simulink model "v_5_IHA_NEW_Plant"  (R2020b)
settings: Solver=VariableStepAuto  StartTime=0.0  StopTime=10  RelTol=1e-3  EnableMultiTasking=on
InitFcn:
  | variables;
values from neighbouring files (symbols this model uses):
  b = 54.2e-6    (= 5.42e-05)    [variables.m]
  d = 1.1e-6    (= 1.1e-06)    [variables.m]
  g = 9.81    [variables.m]
  Ixx = 8.1e-3    (= 0.0081)    [variables.m]
  Iyy = 8.1e-3    (= 0.0081)    [variables.m]
  Izz = 14.2e-3    (= 0.0142)    [variables.m]
  Jr = 104e-6    (= 0.000104)    [variables.m]
  L = 0.24    [variables.m]
  m = 1.0    (= 1)    [variables.m]
  Phi_D = 5    [variables.m]
  Phi_P = 30    [variables.m]
  Psi_D = 5    [variables.m]
  Psi_P = 30    [variables.m]
  Theta_D = 5    [variables.m]
  Theta_P = 30    [variables.m]
  Ts = 0.01    [find_metrics_DQN.m]    (also in v_5_IHA_NEW_Plant_For_DDPG.m; v_5_IHA_NEW_Plant_For_DQN.m)
  Z_D = 12    [variables.m]
  Z_P = 40    [variables.m]
undefined symbols (not defined in the file or in its folder): DiscIntNeverNeededParam
libraries: rllib x4, dspswit3 x4, simulink x3
settings Model: Creator=RafadanTayfa  LastModifiedBy=RafadanTayfa
settings SolverCC: ZeroCrossAlgorithm=Adaptive

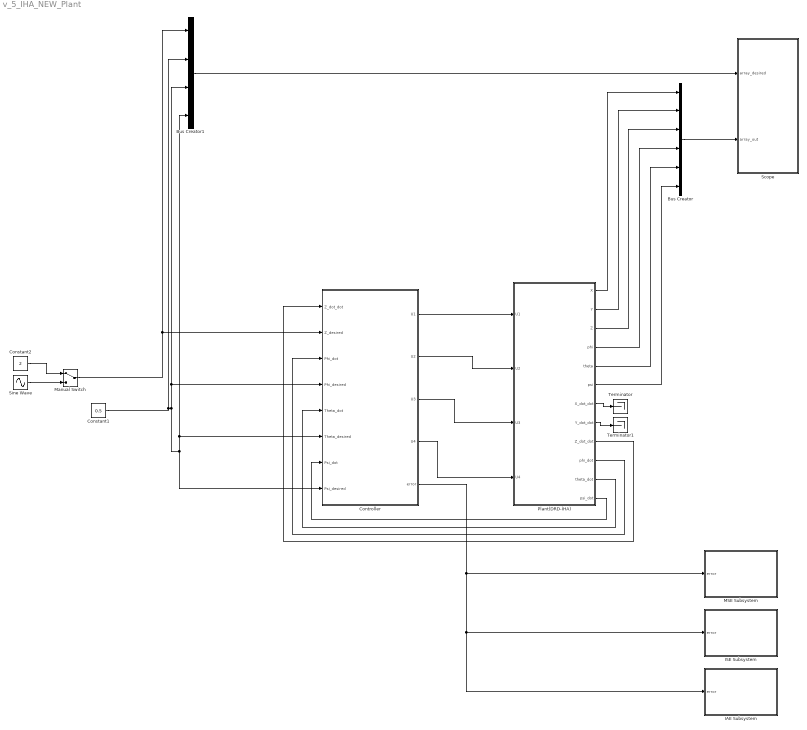
== system v_5_IHA_NEW_Plant ==
  Bus Creator : BusCreator  Inputs=6
  Bus Creator1 : BusCreator  Inputs=4
  Constant1 : Constant  Value=0.5
  Constant2 : Constant  Value=2
  Controller : Subsystem
  IAE Subsystem : Subsystem
  ISE Subsystem : Subsystem
  MSE Subsystem : Subsystem
  Manual Switch : ManualSwitch
  Plant(DRD-İHA) : Subsystem
  Scope : Subsystem
  Sine Wave : Sin  Bias=6  Frequency=pi/2  SampleTime=0
  Terminator : Terminator
  Terminator1 : Terminator
  wires:
  Plant(DRD-İHA)/7(X_dot_dot) -> Terminator/1
  Controller/4(U4) -> Plant(DRD-İHA)/4(U4)
  Controller/3(U3) -> Plant(DRD-İHA)/3(U3)
  Controller/2(U2) -> Plant(DRD-İHA)/2(U2)
  Controller/1(U1) -> Plant(DRD-İHA)/1("U1 ")
  Plant(DRD-İHA)/12(psi_dot) -> Controller/7(Psi_dot)
  Plant(DRD-İHA)/10(phi_dot) -> Controller/3(Phi_dot)
  Plant(DRD-İHA)/11(theta_dot) -> Controller/5(Theta_dot)
  Plant(DRD-İHA)/2(Y) -> Bus Creator/2
  Plant(DRD-İHA)/1(X) -> Bus Creator/1
  Plant(DRD-İHA)/3(Z) -> Bus Creator/3
  Plant(DRD-İHA)/4(phi) -> Bus Creator/4
  Plant(DRD-İHA)/5(theta) -> Bus Creator/5
  Plant(DRD-İHA)/6(psi) -> Bus Creator/6
  Manual Switch/1 -> Bus Creator1/1, Controller/2(Z_desired)
  Constant1/1 -> Bus Creator1/2, Controller/4(Phi_desired), Bus Creator1/3, Controller/6(Theta_desired), Bus Creator1/4, Controller/8(Psi_desired)
  Bus Creator1/1 -> Scope/1(array_desired)
  Bus Creator/1 -> Scope/2(array_out)
  Plant(DRD-İHA)/9(Z_dot_dot) -> Controller/1("Z_dot_dot ")
  Plant(DRD-İHA)/8(Y_dot_dot) -> Terminator1/1
  Controller/5(error) -> MSE Subsystem/1(error), IAE Subsystem/1(error), ISE Subsystem/1(error)
  Constant2/1 -> Manual Switch/1
  Sine Wave/1 -> Manual Switch/2

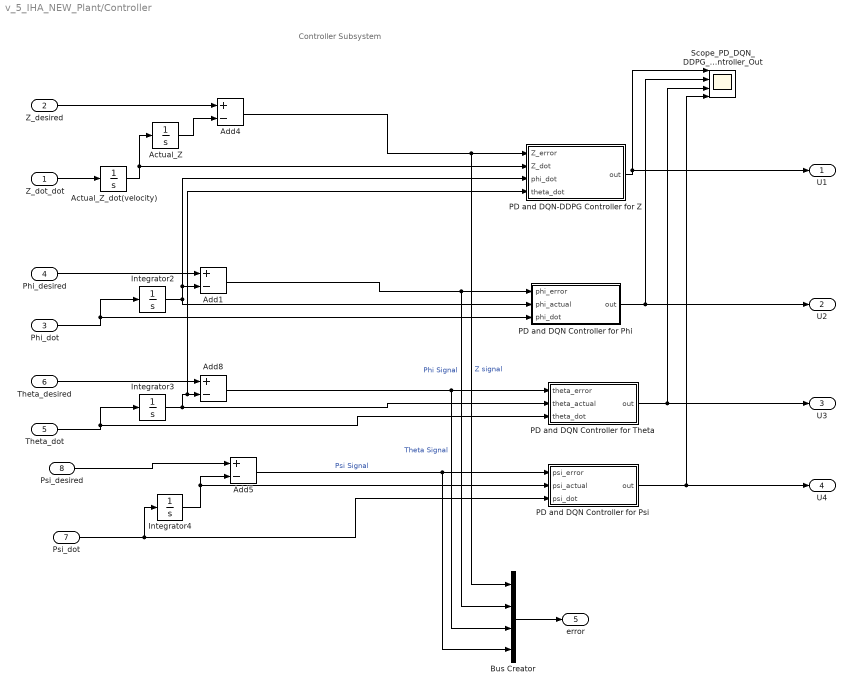
== system v_5_IHA_NEW_Plant/Controller ==
  note: Controller Subsystem
  "Z_dot_dot " : Inport
  Z_desired : Inport  Port=2
  Phi_dot : Inport  Port=3
  Phi_desired : Inport  Port=4
  Theta_dot : Inport  Port=5
  Theta_desired : Inport  Port=6
  Psi_dot : Inport  Port=7
  Psi_desired : Inport  Port=8
  Actual_Z : Integrator  LimitOutput=on  UpperSaturationLimit=800  LowerSaturationLimit=0  ZeroCross=off
  Actual_Z_dot(velocity) : Integrator  ZeroCross=off
  Add{1,4..5,8} (4 alike) : Sum  Inputs=+-
  Bus Creator : BusCreator  Inputs=4
  Integrator2 : Integrator  WrapState=on  ZeroCross=off
  Integrator3 : Integrator  WrapState=on  ZeroCross=off
  Integrator4 : Integrator  WrapState=on  ZeroCross=off
  PD and DQN Controller for Phi : Subsystem
  PD and DQN Controller for Psi : Subsystem
  PD and DQN Controller for Theta : Subsystem
  PD and DQN-DDPG Controller for Z : Subsystem
  Scope_PD_DQN_DDPG_Controller_Out : Scope  NumInputPorts=4
  U1 : Outport
  U2 : Outport  Port=2
  U3 : Outport  Port=3
  U4 : Outport  Port=4
  error : Outport  Port=5
  wires:
  Phi_desired/1 -> Add1/1
  "Z_dot_dot "/1 -> Actual_Z_dot(velocity)/1
  Actual_Z_dot(velocity)/1 -> Actual_Z/1, PD and DQN-DDPG Controller for Z/2(Z_dot)
  Integrator2/1 -> PD and DQN Controller for Phi/2(phi_actual), PD and DQN-DDPG Controller for Z/3(phi_dot), Add1/2
  Add1/1 -> Bus Creator/2, PD and DQN Controller for Phi/1(phi_error)  "Phi Signal"
  Integrator3/1 -> PD and DQN-DDPG Controller for Z/4(theta_dot), Add8/2, PD and DQN Controller for Theta/2(theta_actual)
  Theta_desired/1 -> Add8/1
  Theta_dot/1 -> PD and DQN Controller for Theta/3(theta_dot), Integrator3/1
  Add8/1 -> Bus Creator/3, PD and DQN Controller for Theta/1(theta_error)  "Theta Signal"
  Actual_Z/1 -> Add4/2
  Z_desired/1 -> Add4/1
  Psi_desired/1 -> Add5/1
  Add5/1 -> Bus Creator/4, PD and DQN Controller for Psi/1(psi_error)  "Psi Signal"
  Add4/1 -> Bus Creator/1, PD and DQN-DDPG Controller for Z/1(Z_error)  "Z signal"
  PD and DQN-DDPG Controller for Z/1(out) -> Scope_PD_DQN_DDPG_Controller_Out/1, U1/1
  Phi_dot/1 -> PD and DQN Controller for Phi/3(phi_dot), Integrator2/1
  Psi_dot/1 -> Integrator4/1, PD and DQN Controller for Psi/3(psi_dot)
  Integrator4/1 -> PD and DQN Controller for Psi/2(psi_actual), Add5/2
  Bus Creator/1 -> error/1
  PD and DQN Controller for Phi/1(out) -> U2/1, Scope_PD_DQN_DDPG_Controller_Out/2
  PD and DQN Controller for Theta/1(out) -> U3/1, Scope_PD_DQN_DDPG_Controller_Out/3
  PD and DQN Controller for Psi/1(out) -> U4/1, Scope_PD_DQN_DDPG_Controller_Out/4

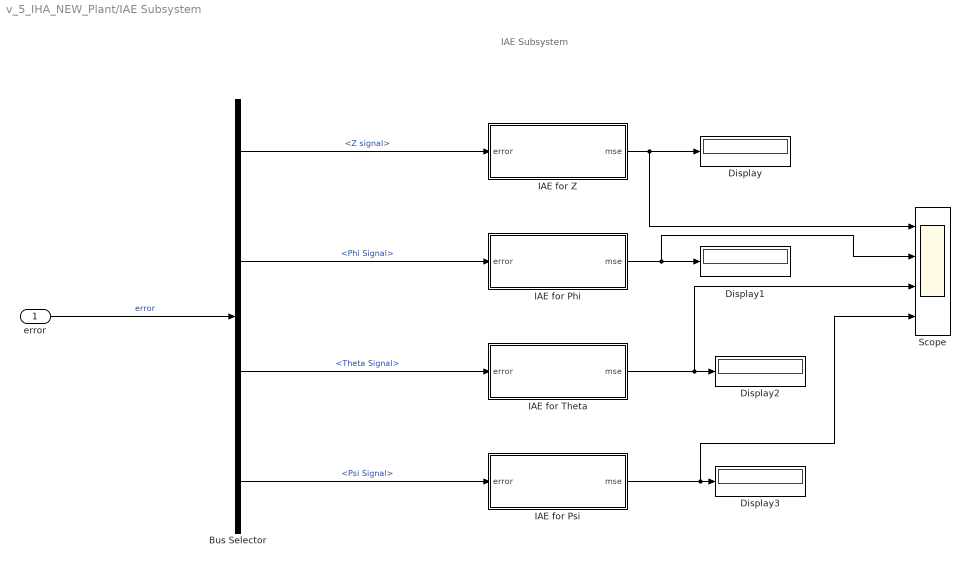
== system v_5_IHA_NEW_Plant/IAE Subsystem ==
  note: IAE Subsystem
  error : Inport
  Bus Selector : BusSelector  OutputSignals=Z signal,Phi Signal,Theta Signal,Psi Signal
  Display{,1..3} (4 alike) : Display
  IAE for Phi : Subsystem
  IAE for Psi : Subsystem
  IAE for Theta : Subsystem
  IAE for Z : Subsystem
  Scope : Scope  NumInputPorts=4
  wires:
  IAE for Z/1(mse) -> Scope/1, Display/1
  error/1 -> Bus Selector/1  "error"
  Bus Selector/1 -> IAE for Z/1(error)  "<Z signal>"
  IAE for Phi/1(mse) -> Scope/2, Display1/1
  Bus Selector/2 -> IAE for Phi/1(error)  "<Phi Signal>"
  Bus Selector/3 -> IAE for Theta/1(error)  "<Theta Signal>"
  Bus Selector/4 -> IAE for Psi/1(error)  "<Psi Signal>"
  IAE for Theta/1(mse) -> Scope/3, Display2/1
  IAE for Psi/1(mse) -> Scope/4, Display3/1

== system v_5_IHA_NEW_Plant/ISE Subsystem ==
  note: ISE Subsystem
  error : Inport
  Bus Selector : BusSelector  OutputSignals=Z signal,Phi Signal,Theta Signal,Psi Signal
  Display{,1..3} (4 alike) : Display
  ISE for Phi : Subsystem
  ISE for Psi : Subsystem
  ISE for Theta : Subsystem
  ISE for Z : Subsystem
  Scope : Scope  NumInputPorts=4
  wires:
  ISE for Psi/1(mse) -> Display3/1, Scope/4
  ISE for Theta/1(mse) -> Display2/1, Scope/3
  Bus Selector/4 -> ISE for Psi/1(error)  "<Psi Signal>"
  Bus Selector/3 -> ISE for Theta/1(error)  "<Theta Signal>"
  Bus Selector/2 -> ISE for Phi/1(error)  "<Phi Signal>"
  ISE for Phi/1(mse) -> Display1/1, Scope/2
  Bus Selector/1 -> ISE for Z/1(error)  "<Z signal>"
  error/1 -> Bus Selector/1  "error"
  ISE for Z/1(mse) -> Display/1, Scope/1

== system v_5_IHA_NEW_Plant/MSE Subsystem ==
  note: MSE Subsystem
  error : Inport
  Bus Selector : BusSelector  OutputSignals=Z signal,Phi Signal,Theta Signal,Psi Signal
  Display{,1..3} (4 alike) : Display
  MSE for Phi : Subsystem
  MSE for Psi : Subsystem
  MSE for Theta : Subsystem
  MSE for Z : Subsystem
  Scope : Scope  NumInputPorts=4
  wires:
  MSE for Z/1(mse) -> Scope/1, Display/1
  error/1 -> Bus Selector/1  "error"
  Bus Selector/1 -> MSE for Z/1(error)  "<Z signal>"
  MSE for Phi/1(mse) -> Scope/2, Display1/1
  Bus Selector/2 -> MSE for Phi/1(error)  "<Phi Signal>"
  Bus Selector/3 -> MSE for Theta/1(error)  "<Theta Signal>"
  Bus Selector/4 -> MSE for Psi/1(error)  "<Psi Signal>"
  MSE for Theta/1(mse) -> Scope/3, Display2/1
  MSE for Psi/1(mse) -> Scope/4, Display3/1

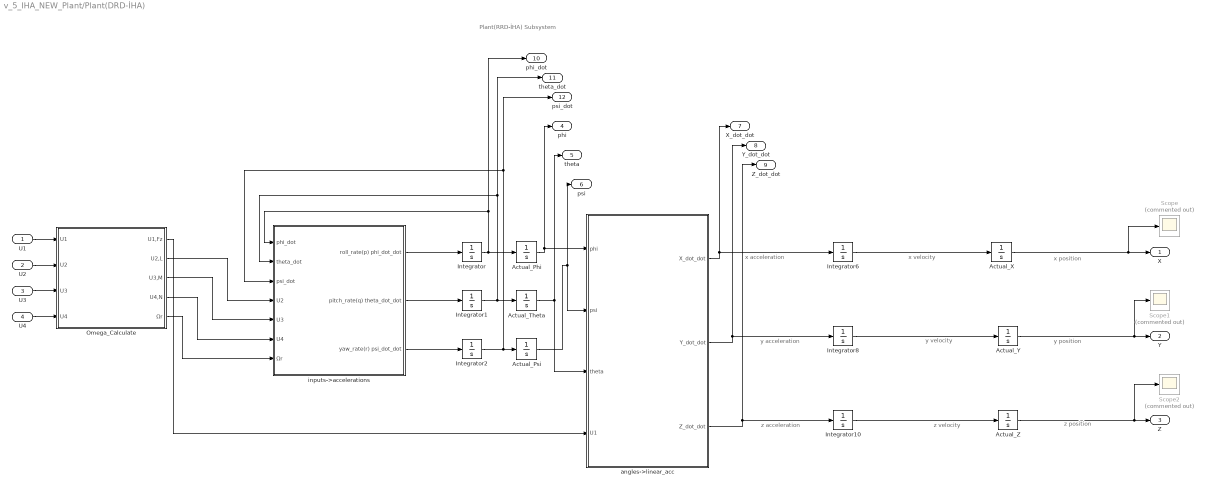
== system v_5_IHA_NEW_Plant/Plant(DRD-İHA) ==
  note: Plant(RRD-İHA) Subsystem
  note: z position
  note: y position
  note: x position
  note: z velocity
  note: y velocity
  note: x velocity
  note: z acceleration
  note: y acceleration
  note: x acceleration
  "U1 " : Inport
  U2 : Inport  Port=2
  U3 : Inport  Port=3
  U4 : Inport  Port=4
  Actual_Phi : Integrator  WrapState=on  ZeroCross=off
  Actual_Psi : Integrator  WrapState=on  ZeroCross=off
  Actual_Theta : Integrator  WrapState=on  ZeroCross=off
  Actual_X : Integrator  ZeroCross=off
  Actual_Y : Integrator  ZeroCross=off
  Actual_Z : Integrator  LimitOutput=on  UpperSaturationLimit=800  LowerSaturationLimit=0  ZeroCross=off
  Integrator{,1..2,6,10} (5 alike) : Integrator  ZeroCross=off
  Integrator8 : Integrator  UpperSaturationLimit=0  ZeroCross=off
  "Omega_Calculate " : Subsystem
  Scope : Scope  Commented=on
  Scope1 : Scope  Commented=on
  Scope2 : Scope  Commented=on
  angles->linear_acc : Subsystem
  inputs->accelerations : Subsystem
  X : Outport
  Y : Outport  Port=2
  Z : Outport  Port=3
  phi : Outport  Port=4
  theta : Outport  Port=5
  psi : Outport  Port=6
  X_dot_dot : Outport  Port=7
  Y_dot_dot : Outport  Port=8
  Z_dot_dot : Outport  Port=9
  phi_dot : Outport  Port=10
  theta_dot : Outport  Port=11
  psi_dot : Outport  Port=12
  wires:
  Integrator6/1 -> Actual_X/1
  angles->linear_acc/3(Z_dot_dot) -> Z_dot_dot/1, Integrator10/1
  Integrator8/1 -> Actual_Y/1
  Actual_Z/1 -> Scope2/1, Z/1
  "Omega_Calculate "/1(U1,Fz) -> angles->linear_acc/4(U1)
  Integrator2/1 -> psi_dot/1, inputs->accelerations/3(psi_dot), Actual_Psi/1
  Integrator10/1 -> Actual_Z/1
  Actual_Theta/1 -> theta/1, angles->linear_acc/3(theta)
  Actual_Y/1 -> Scope1/1, Y/1
  Integrator/1 -> phi_dot/1, inputs->accelerations/1(phi_dot), Actual_Phi/1
  Actual_X/1 -> Scope/1, X/1
  Actual_Phi/1 -> phi/1, angles->linear_acc/1(phi)
  Integrator1/1 -> theta_dot/1, inputs->accelerations/2(theta_dot), Actual_Theta/1
  Actual_Psi/1 -> psi/1, angles->linear_acc/2(psi)
  angles->linear_acc/1(X_dot_dot) -> X_dot_dot/1, Integrator6/1
  "Omega_Calculate "/2("U2,L ") -> inputs->accelerations/4(U2)
  "Omega_Calculate "/3(U3,M) -> inputs->accelerations/5(U3)
  "Omega_Calculate "/4("U4,N ") -> inputs->accelerations/6(U4)
  "Omega_Calculate "/5(Ωr) -> inputs->accelerations/7(Ωr)
  angles->linear_acc/2(Y_dot_dot) -> Y_dot_dot/1, Integrator8/1
  inputs->accelerations/2(pitch_rate(q) theta_dot_dot) -> Integrator1/1
  inputs->accelerations/1(roll_rate(p) phi_dot_dot) -> Integrator/1
  inputs->accelerations/3(yaw_rate(r) psi_dot_dot) -> Integrator2/1
  "U1 "/1 -> "Omega_Calculate "/1(U1)
  U2/1 -> "Omega_Calculate "/2(U2)
  U3/1 -> "Omega_Calculate "/3(U3)
  U4/1 -> "Omega_Calculate "/4(U4)

== system v_5_IHA_NEW_Plant/Scope ==
  note: Scope Subsystem
  array_desired : Inport
  array_out : Inport  Port=2
  Scope_Phi : Scope
  Scope_Psi : Scope
  Scope_Theta : Scope
  Scope_X : Scope
  Scope_Y : Scope
  Scope_Z : Scope
  array2array : MATLAB Function  TreatAsAtomicUnit=on
  wires:
  array_out/1 -> array2array/2(array_out)
  array_desired/1 -> array2array/1(array_desired)
  array2array/1(X_array) -> Scope_X/1
  array2array/2(Y_array) -> Scope_Y/1
  array2array/3(Z_array) -> Scope_Z/1
  array2array/4(Phi_array) -> Scope_Phi/1
  array2array/5(Theta_array) -> Scope_Theta/1
  array2array/6(Psi_array) -> Scope_Psi/1

== system v_5_IHA_NEW_Plant/Controller/PD and DQN Controller for Phi ==
  note: PD and DQN Controller Subsystem
  phi_error : Inport
  phi_actual : Inport  Port=2
  phi_dot : Inport  Port=3
  DQN Controller for Phi : Subsystem  Commented=on  TreatAsAtomicUnit=on
  PD Controller for Phi Angle : Subsystem  TreatAsAtomicUnit=on
  out : Outport
  wires:
  phi_dot/1 -> PD Controller for Phi Angle/3(phi_dot)
  phi_actual/1 -> PD Controller for Phi Angle/2(phi_actual)
  phi_error/1 -> PD Controller for Phi Angle/1(phi_error)
  PD Controller for Phi Angle/1(out) -> out/1

== system v_5_IHA_NEW_Plant/Controller/PD and DQN Controller for Psi ==
  note: PD and DQN-DDPG Controller Subsystem
  psi_error : Inport
  psi_actual : Inport  Port=2
  psi_dot : Inport  Port=3
  DQN-DDPG Controller for Psi : Subsystem  Commented=on  TreatAsAtomicUnit=on
  PD Controller for Psi Angle : Subsystem  TreatAsAtomicUnit=on
  out : Outport
  wires:
  psi_error/1 -> PD Controller for Psi Angle/1(psi_error)
  psi_actual/1 -> PD Controller for Psi Angle/2(psi_actual)
  psi_dot/1 -> PD Controller for Psi Angle/3(psi_dot)
  PD Controller for Psi Angle/1(out) -> out/1

== system v_5_IHA_NEW_Plant/Controller/PD and DQN Controller for Theta ==
  note: PD and DQN-DDPG Controller Subsystem
  theta_error : Inport
  theta_actual : Inport  Port=2
  theta_dot : Inport  Port=3
  DQN-DDPG Controller for Theta : Subsystem  Commented=on  TreatAsAtomicUnit=on
  PD Controller for Theta Angle : Subsystem  TreatAsAtomicUnit=on
  out : Outport
  wires:
  theta_error/1 -> PD Controller for Theta Angle/1(theta_error)
  theta_actual/1 -> PD Controller for Theta Angle/2(theta_actual)
  theta_dot/1 -> PD Controller for Theta Angle/3(theta_dot)
  PD Controller for Theta Angle/1(out) -> out/1

== system v_5_IHA_NEW_Plant/Controller/PD and DQN-DDPG Controller for Z ==
  note: PD and DQN-DDPG Controller Subsystem
  Z_error : Inport
  Z_dot : Inport  Port=2
  phi_dot : Inport  Port=3
  theta_dot : Inport  Port=4
  DQN-DDPG Controller for Z : Subsystem  Commented=on  TreatAsAtomicUnit=on
  PD Controller for Z : Subsystem  TreatAsAtomicUnit=on
  out : Outport
  wires:
  phi_dot/1 -> PD Controller for Z/3(phi_dot)
  theta_dot/1 -> PD Controller for Z/4(theta_dot)
  Z_error/1 -> PD Controller for Z/1(Z_error)
  Z_dot/1 -> PD Controller for Z/2(Z_dot)
  PD Controller for Z/1(out) -> out/1

== system v_5_IHA_NEW_Plant/IAE Subsystem/IAE for Phi ==
  note: IAE for Phi
  error : Inport
  Add : Sum
  Delay : Delay  DelayLength=1
  error2abs : MATLAB Function  TreatAsAtomicUnit=on
  mse : Outport
  wires:
  Add/1 -> mse/1, Delay/1
  Delay/1 -> Add/1
  error2abs/1(abs) -> Add/2
  error/1 -> error2abs/1(error)

== system v_5_IHA_NEW_Plant/IAE Subsystem/IAE for Psi ==
  note: IAE for Psi
  error : Inport
  Add : Sum
  Delay : Delay  DelayLength=1
  error2abs : MATLAB Function  TreatAsAtomicUnit=on
  mse : Outport
  wires:
  error/1 -> error2abs/1(error)
  error2abs/1(abs) -> Add/2
  Add/1 -> mse/1, Delay/1
  Delay/1 -> Add/1

== system v_5_IHA_NEW_Plant/IAE Subsystem/IAE for Theta ==
  note: IAE for Theta
  error : Inport
  Add : Sum
  Delay : Delay  DelayLength=1
  error2abs : MATLAB Function  TreatAsAtomicUnit=on
  mse : Outport
  wires:
  Delay/1 -> Add/1
  Add/1 -> mse/1, Delay/1
  error/1 -> error2abs/1(error)
  error2abs/1(abs) -> Add/2

== system v_5_IHA_NEW_Plant/IAE Subsystem/IAE for Z ==
  note: IAE for Z
  error : Inport
  Add : Sum
  Delay : Delay  DelayLength=1
  error2abs : MATLAB Function  TreatAsAtomicUnit=on
  mse : Outport
  wires:
  Delay/1 -> Add/1
  Add/1 -> mse/1, Delay/1
  error2abs/1(abs) -> Add/2
  error/1 -> error2abs/1(error)

== system v_5_IHA_NEW_Plant/ISE Subsystem/ISE for Phi ==
  note: ISE for Phi
  error : Inport
  Add : Sum
  Delay : Delay  DelayLength=1
  Square1 : Math  Operator=square  SaturateOnIntegerOverflow=on
  mse : Outport
  wires:
  Delay/1 -> Add/1
  Add/1 -> Delay/1, mse/1
  Square1/1 -> Add/2
  error/1 -> Square1/1

== system v_5_IHA_NEW_Plant/ISE Subsystem/ISE for Psi ==
  note: ISE for Psi
  error : Inport
  Add : Sum
  Delay : Delay  DelayLength=1
  Square1 : Math  Operator=square  SaturateOnIntegerOverflow=on
  mse : Outport
  wires:
  Delay/1 -> Add/1
  Add/1 -> Delay/1, mse/1
  Square1/1 -> Add/2
  error/1 -> Square1/1

== system v_5_IHA_NEW_Plant/ISE Subsystem/ISE for Theta ==
  note: ISE for Theta
  error : Inport
  Add : Sum
  Delay : Delay  DelayLength=1
  Square1 : Math  Operator=square  SaturateOnIntegerOverflow=on
  mse : Outport
  wires:
  error/1 -> Square1/1
  Square1/1 -> Add/2
  Add/1 -> Delay/1, mse/1
  Delay/1 -> Add/1

== system v_5_IHA_NEW_Plant/ISE Subsystem/ISE for Z ==
  note: ISE for Z
  error : Inport
  Add : Sum
  Delay : Delay  DelayLength=1
  Square1 : Math  Operator=square  SaturateOnIntegerOverflow=on
  mse : Outport
  wires:
  error/1 -> Square1/1
  Square1/1 -> Add/2
  Add/1 -> Delay/1, mse/1
  Delay/1 -> Add/1

== system v_5_IHA_NEW_Plant/MSE Subsystem/MSE for Phi ==
  note: MSE for Phi
  error : Inport
  Add : Sum
  Counter1 : dspswit3/Counter  Direction=Up  CountEvent=Free running  CounterSize=32 bits  MaxCount=255  InitialCount=1  Output=Count  HitValue=32  ResetInput=off  SamplesPerFrame=1  Ts=Ts  CntDtype=double  HitDtype=Logical
  Delay : Delay  DelayLength=1
  Divide : Product  Inputs=*/
  Square1 : Math  Operator=square  SaturateOnIntegerOverflow=on
  mse : Outport
  wires:
  Counter1/1 -> Divide/2
  error/1 -> Square1/1
  Square1/1 -> Add/2
  Divide/1 -> mse/1
  Add/1 -> Delay/1, Divide/1
  Delay/1 -> Add/1

== system v_5_IHA_NEW_Plant/MSE Subsystem/MSE for Psi ==
  error : Inport
  Add : Sum
  Counter1 : dspswit3/Counter  Direction=Up  CountEvent=Free running  CounterSize=32 bits  MaxCount=255  InitialCount=1  Output=Count  HitValue=32  ResetInput=off  SamplesPerFrame=1  Ts=Ts  CntDtype=double  HitDtype=Logical
  Delay : Delay  DelayLength=1
  Divide : Product  Inputs=*/
  Square1 : Math  Operator=square  SaturateOnIntegerOverflow=on
  mse : Outport
  wires:
  Counter1/1 -> Divide/2
  error/1 -> Square1/1
  Square1/1 -> Add/2
  Divide/1 -> mse/1
  Add/1 -> Delay/1, Divide/1
  Delay/1 -> Add/1

== system v_5_IHA_NEW_Plant/MSE Subsystem/MSE for Theta ==
  error : Inport
  Add : Sum
  Counter1 : dspswit3/Counter  Direction=Up  CountEvent=Free running  CounterSize=32 bits  MaxCount=255  InitialCount=1  Output=Count  HitValue=32  ResetInput=off  SamplesPerFrame=1  Ts=Ts  CntDtype=double  HitDtype=Logical
  Delay : Delay  DelayLength=1
  Divide : Product  Inputs=*/
  Square1 : Math  Operator=square  SaturateOnIntegerOverflow=on
  mse : Outport
  wires:
  Delay/1 -> Add/1
  Add/1 -> Delay/1, Divide/1
  Divide/1 -> mse/1
  Square1/1 -> Add/2
  error/1 -> Square1/1
  Counter1/1 -> Divide/2

== system v_5_IHA_NEW_Plant/MSE Subsystem/MSE for Z ==
  error : Inport
  Add : Sum
  Counter1 : dspswit3/Counter  Direction=Up  CountEvent=Free running  CounterSize=32 bits  MaxCount=255  InitialCount=1  Output=Count  HitValue=32  ResetInput=off  SamplesPerFrame=1  Ts=Ts  CntDtype=double  HitDtype=Logical
  Delay : Delay  DelayLength=1
  Divide : Product  Inputs=*/
  Square1 : Math  Operator=square  SaturateOnIntegerOverflow=on
  mse : Outport
  wires:
  Delay/1 -> Add/1
  Add/1 -> Delay/1, Divide/1
  Divide/1 -> mse/1
  Square1/1 -> Add/2
  error/1 -> Square1/1
  Counter1/1 -> Divide/2

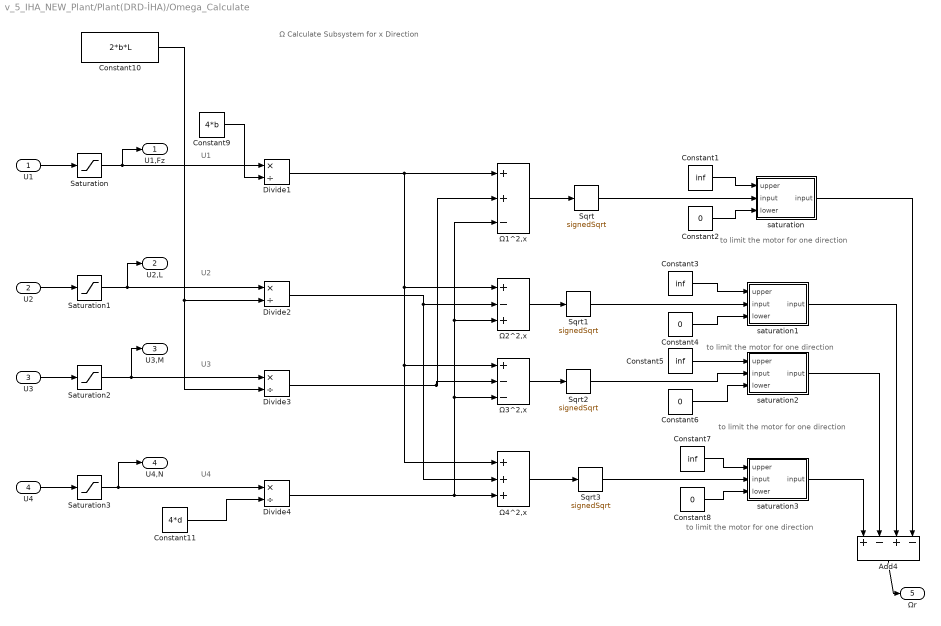
== system v_5_IHA_NEW_Plant/Plant(DRD-İHA)/Omega_Calculate  ==
  note: to limit the motor for one direction
  note: Ω Calculate Subsystem for x Direction
  note: U1
  note: U2
  note: U3
  note: U4
  note: to limit the motor for one direction
  note: to limit the motor for one direction
  note: to limit the motor for one direction
  U1 : Inport
  U2 : Inport  Port=2
  U3 : Inport  Port=3
  U4 : Inport  Port=4
  Add4 : Sum  Inputs=+-+-
  Constant{1,3,5,7} (4 alike) : Constant  Value=inf
  Constant10 : Constant  Value=2*b*L
  Constant11 : Constant  Value=4*d
  Constant{2,4,6,8} (4 alike) : Constant  Value=0
  Constant9 : Constant  Value=4*b
  Divide{1..4} (4 alike) : Product  Inputs=*/
  Saturation : Saturate  UpperLimit=15.7  LowerLimit=0
  Saturation1 : Saturate  UpperLimit=1  LowerLimit=-1
  Saturation2 : Saturate  UpperLimit=1  LowerLimit=-1
  Saturation3 : Saturate  UpperLimit=1  LowerLimit=-1
  Sqrt{,1..3} (4 alike) : Sqrt  Operator=signedSqrt  SaturateOnIntegerOverflow=on
  saturation : MATLAB Function  TreatAsAtomicUnit=on
  saturation1 : MATLAB Function  TreatAsAtomicUnit=on
  saturation2 : MATLAB Function  TreatAsAtomicUnit=on
  saturation3 : MATLAB Function  TreatAsAtomicUnit=on
  Ω1^2,x : Sum  Inputs=++-
  Ω2^2,x : Sum  Inputs=+-+
  Ω3^2,x : Sum  Inputs=+--
  Ω4^2,x : Sum  Inputs=+++
  U1,Fz : Outport
  "U2,L " : Outport  Port=2
  U3,M : Outport  Port=3
  "U4,N " : Outport  Port=4
  Ωr : Outport  Port=5
  wires:
  saturation2/1(input) -> Add4/2
  saturation3/1(input) -> Add4/1
  saturation/1(input) -> Add4/4
  saturation1/1(input) -> Add4/3
  Add4/1 -> Ωr/1
  Constant1/1 -> saturation/1(upper)
  Constant2/1 -> saturation/3(lower)
  Constant4/1 -> saturation1/3(lower)
  Constant3/1 -> saturation1/1(upper)
  Constant6/1 -> saturation2/3(lower)
  Constant5/1 -> saturation2/1(upper)
  Constant8/1 -> saturation3/3(lower)
  Constant7/1 -> saturation3/1(upper)
  Divide3/1 -> Ω3^2,x/2, Ω1^2,x/2
  Divide1/1 -> Ω3^2,x/1, Ω4^2,x/1, Ω2^2,x/1, Ω1^2,x/1
  Divide2/1 -> Ω4^2,x/2, Ω2^2,x/2
  Divide4/1 -> Ω1^2,x/3, Ω2^2,x/3, Ω3^2,x/3, Ω4^2,x/3
  Ω3^2,x/1 -> Sqrt2/1
  Constant11/1 -> Divide4/2
  Constant10/1 -> Divide2/2, Divide3/2
  Ω1^2,x/1 -> Sqrt/1
  Ω4^2,x/1 -> Sqrt3/1
  Ω2^2,x/1 -> Sqrt1/1
  Constant9/1 -> Divide1/2
  Sqrt/1 -> saturation/2("input ")
  Sqrt1/1 -> saturation1/2("input ")
  Sqrt2/1 -> saturation2/2("input ")
  Sqrt3/1 -> saturation3/2("input ")
  U1/1 -> Saturation/1
  U2/1 -> Saturation1/1
  U3/1 -> Saturation2/1
  U4/1 -> Saturation3/1
  Saturation/1 -> U1,Fz/1, Divide1/1
  Saturation1/1 -> "U2,L "/1, Divide2/1
  Saturation2/1 -> U3,M/1, Divide3/1
  Saturation3/1 -> "U4,N "/1, Divide4/1

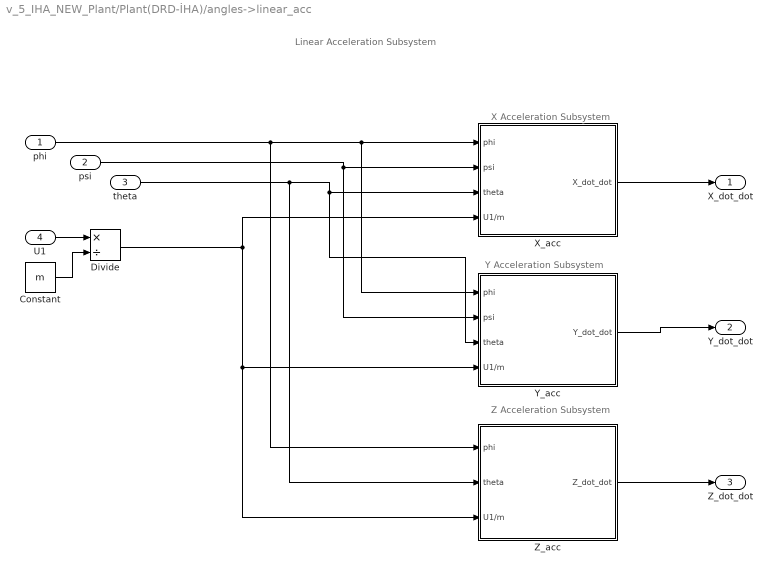
== system v_5_IHA_NEW_Plant/Plant(DRD-İHA)/angles->linear_acc ==
  note: Linear Acceleration Subsystem
  note: X Acceleration Subsystem
  note: Y Acceleration Subsystem
  note: Z Acceleration Subsystem
  phi : Inport
  psi : Inport  Port=2
  theta : Inport  Port=3
  U1 : Inport  Port=4
  Constant : Constant  Value=m
  Divide : Product  Inputs=*/
  X_acc : Subsystem
  Y_acc : Subsystem
  Z_acc : Subsystem
  X_dot_dot : Outport
  Y_dot_dot : Outport  Port=2
  Z_dot_dot : Outport  Port=3
  wires:
  phi/1 -> Z_acc/1(phi), Y_acc/1(phi), X_acc/1(phi)
  psi/1 -> Y_acc/2(psi), X_acc/2(psi)
  theta/1 -> Y_acc/3(theta), X_acc/3(theta), Z_acc/2(theta)
  U1/1 -> Divide/1
  Constant/1 -> Divide/2
  Divide/1 -> Z_acc/3(U1/m), Y_acc/4(U1/m), X_acc/4(U1/m)
  X_acc/1("X_dot_dot\t") -> X_dot_dot/1
  Y_acc/1("Y_dot_dot\t") -> Y_dot_dot/1
  Z_acc/1("Z_dot_dot\t") -> Z_dot_dot/1

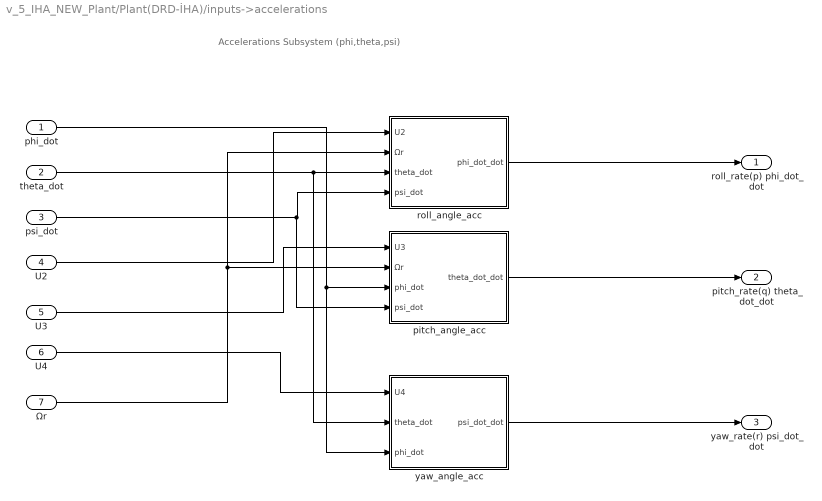
== system v_5_IHA_NEW_Plant/Plant(DRD-İHA)/inputs->accelerations ==
  note: Accelerations Subsystem (phi,theta,psi)
  phi_dot : Inport
  theta_dot : Inport  Port=2
  psi_dot : Inport  Port=3
  U2 : Inport  Port=4
  U3 : Inport  Port=5
  U4 : Inport  Port=6
  Ωr : Inport  Port=7
  pitch_angle_acc : Subsystem
  roll_angle_acc : Subsystem
  yaw_angle_acc : Subsystem
  roll_rate(p) phi_dot_dot : Outport
  pitch_rate(q) theta_dot_dot : Outport  Port=2
  yaw_rate(r) psi_dot_dot : Outport  Port=3
  wires:
  roll_angle_acc/1(phi_dot_dot) -> roll_rate(p) phi_dot_dot/1
  pitch_angle_acc/1(theta_dot_dot) -> pitch_rate(q) theta_dot_dot/1
  yaw_angle_acc/1(psi_dot_dot) -> yaw_rate(r) psi_dot_dot/1
  phi_dot/1 -> yaw_angle_acc/3(phi_dot), pitch_angle_acc/3(phi_dot)
  theta_dot/1 -> yaw_angle_acc/2(theta_dot), roll_angle_acc/3(theta_dot)
  psi_dot/1 -> pitch_angle_acc/4(psi_dot), roll_angle_acc/4(psi_dot)
  U2/1 -> roll_angle_acc/1(U2)
  U3/1 -> pitch_angle_acc/1(U3)
  U4/1 -> yaw_angle_acc/1(U4)
  Ωr/1 -> roll_angle_acc/2(Ωr), pitch_angle_acc/2(Ωr)

== system v_5_IHA_NEW_Plant/Controller/PD and DQN Controller for Phi/DQN Controller for Phi ==
  Z_error : Inport
  Z_actual : Inport  Port=2
  Z_dot : Inport  Port=3
  DQN Controller : Subsystem  Commented=on
  Terminator : Terminator
  out : Outport
  wires:
  DQN Controller/1(action) -> out/1
  Z_dot/1 -> Terminator/1
  Z_actual/1 -> DQN Controller/2(Z_actual)
  Z_error/1 -> DQN Controller/1(Z_error)

== system v_5_IHA_NEW_Plant/Controller/PD and DQN Controller for Phi/PD Controller for Phi Angle ==
  note: PD Controller for Phi Angle
  phi_error : Inport
  phi_actual : Inport  Port=2
  phi_dot : Inport  Port=3
  Add1 : Sum  Inputs=+-
  Ixx : Gain  Gain=Ixx
  Phi Derivative : Gain  Gain=Phi_D
  Phi Proportional : Gain  Gain=Phi_P
  Terminator : Terminator
  out : Outport
  wires:
  phi_actual/1 -> Terminator/1
  Phi Proportional/1 -> Add1/1
  Ixx/1 -> out/1
  Add1/1 -> Ixx/1
  Phi Derivative/1 -> Add1/2
  phi_dot/1 -> Phi Derivative/1
  phi_error/1 -> Phi Proportional/1

== system v_5_IHA_NEW_Plant/Controller/PD and DQN Controller for Psi/DQN-DDPG Controller for Psi ==
  Z_error : Inport
  Z_actual : Inport  Port=2
  Z_dot : Inport  Port=3
  DQN Controller : Subsystem  Commented=on
  Terminator : Terminator
  out : Outport
  wires:
  Z_error/1 -> DQN Controller/1(Z_error)
  Z_actual/1 -> DQN Controller/2(Z_actual)
  Z_dot/1 -> Terminator/1
  DQN Controller/1(action) -> out/1

== system v_5_IHA_NEW_Plant/Controller/PD and DQN Controller for Psi/PD Controller for Psi Angle ==
  note: PD Controller for Psi Angle
  psi_error : Inport
  psi_actual : Inport  Port=2
  psi_dot : Inport  Port=3
  Add2 : Sum  Inputs=+-
  Izz : Gain  Gain=Izz
  Psi Derivative : Gain  Gain=Psi_D
  Psi Proportional : Gain  Gain=Psi_P
  Terminator : Terminator
  out : Outport
  wires:
  psi_actual/1 -> Terminator/1
  Psi Derivative/1 -> Add2/2
  Add2/1 -> Izz/1
  Psi Proportional/1 -> Add2/1
  psi_error/1 -> Psi Proportional/1
  Izz/1 -> out/1
  psi_dot/1 -> Psi Derivative/1

== system v_5_IHA_NEW_Plant/Controller/PD and DQN Controller for Theta/DQN-DDPG Controller for Theta ==
  Z_error : Inport
  Z_actual : Inport  Port=2
  Z_dot : Inport  Port=3
  DQN Controller : Subsystem  Commented=on
  Terminator : Terminator
  out : Outport
  wires:
  Z_error/1 -> DQN Controller/1(Z_error)
  Z_actual/1 -> DQN Controller/2(Z_actual)
  Z_dot/1 -> Terminator/1
  DQN Controller/1(action) -> out/1

== system v_5_IHA_NEW_Plant/Controller/PD and DQN Controller for Theta/PD Controller for Theta Angle ==
  note: PD Controller for Theta Angle
  theta_error : Inport
  theta_actual : Inport  Port=2
  theta_dot : Inport  Port=3
  Add2 : Sum  Inputs=+-
  Iyy : Gain  Gain=Iyy
  Terminator : Terminator
  Theta Derivative : Gain  Gain=Theta_D
  Theta Proportional : Gain  Gain=Theta_P
  out : Outport
  wires:
  Iyy/1 -> out/1
  theta_actual/1 -> Terminator/1
  theta_dot/1 -> Theta Derivative/1
  theta_error/1 -> Theta Proportional/1
  Theta Derivative/1 -> Add2/2
  Theta Proportional/1 -> Add2/1
  Add2/1 -> Iyy/1

== system v_5_IHA_NEW_Plant/Controller/PD and DQN-DDPG Controller for Z/DQN-DDPG Controller for Z ==
  note: DQN-DDPG Controller for Z
  Z_error : Inport
  Z_dot : Inport  Port=2
  Actual_Z : Integrator  LimitOutput=on  UpperSaturationLimit=800  LowerSaturationLimit=0  ZeroCross=off
  Display : Display
  Observation : Subsystem
  RL Agent : rllib/RL Agent  Agent=saved_agent  ProvideReward=on  ProvideIsDone=on  ProvideCumRwd=off  TreatAsDirectFeedthrough=on  CollectLoggedSignals=on  CollectModelStates=on
  Reward : Subsystem
  Sum : Sum
  Theta_limit_penalty : Subsystem
  out : Outport
  wires:
  Z_dot/1 -> Actual_Z/1
  RL Agent/1 -> out/1
  Theta_limit_penalty/1(reward) -> Sum/2
  Reward/1(reward) -> Sum/1
  Theta_limit_penalty/2(stop) -> RL Agent/3
  Sum/1 -> RL Agent/2
  Z_error/1 -> Observation/1(error), Theta_limit_penalty/1(error), Reward/1(error)
  Observation/1(observation) -> Display/1, RL Agent/1
  Actual_Z/1 -> Observation/2(Actual_Z)

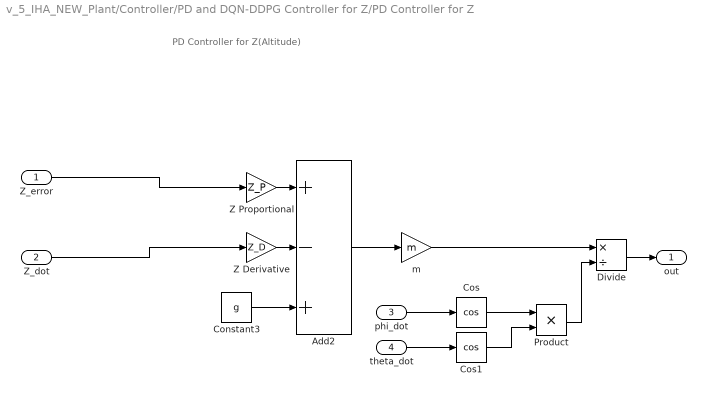
== system v_5_IHA_NEW_Plant/Controller/PD and DQN-DDPG Controller for Z/PD Controller for Z ==
  note: PD Controller for Z(Altitude)
  Z_error : Inport
  Z_dot : Inport  Port=2
  phi_dot : Inport  Port=3
  theta_dot : Inport  Port=4
  Add2 : Sum  Inputs=+-+
  Constant3 : Constant  Value=g
  Cos : Trigonometry  Operator=cos
  Cos1 : Trigonometry  Operator=cos
  Divide : Product  Inputs=*/
  Product : Product
  Z Derivative : Gain  Gain=Z_D
  Z Proportional : Gain  Gain=Z_P
  m : Gain  Gain=m
  out : Outport
  wires:
  Z Derivative/1 -> Add2/2
  Constant3/1 -> Add2/3
  Z_error/1 -> Z Proportional/1
  m/1 -> Divide/1
  Z Proportional/1 -> Add2/1
  Add2/1 -> m/1
  Z_dot/1 -> Z Derivative/1
  Cos/1 -> Product/1
  Product/1 -> Divide/2
  Cos1/1 -> Product/2
  Divide/1 -> out/1
  phi_dot/1 -> Cos/1
  theta_dot/1 -> Cos1/1

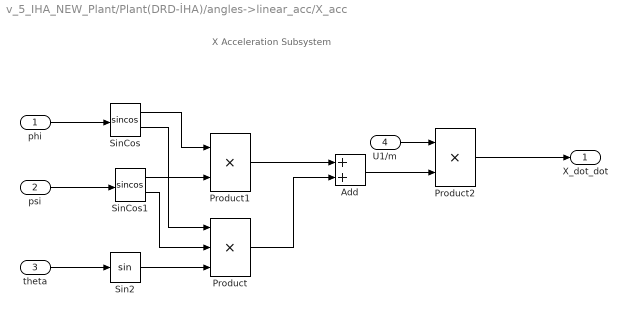
== system v_5_IHA_NEW_Plant/Plant(DRD-İHA)/angles->linear_acc/X_acc ==
  note: X Acceleration Subsystem
  phi : Inport
  psi : Inport  Port=2
  theta : Inport  Port=3
  U1/m : Inport  Port=4
  Add : Sum
  Product : Product  Inputs=3
  Product1 : Product
  Product2 : Product
  Sin2 : Trigonometry
  SinCos : Trigonometry  Operator=sincos
  SinCos1 : Trigonometry  Operator=sincos
  "X_dot_dot\t" : Outport
  wires:
  phi/1 -> SinCos/1
  psi/1 -> SinCos1/1
  theta/1 -> Sin2/1
  SinCos1/2 -> Product/2
  Sin2/1 -> Product/3
  SinCos/1 -> Product1/1
  Product1/1 -> Add/1
  Product/1 -> Add/2
  Add/1 -> Product2/2
  Product2/1 -> "X_dot_dot\t"/1
  U1/m/1 -> Product2/1
  SinCos1/1 -> Product1/2
  SinCos/2 -> Product/1

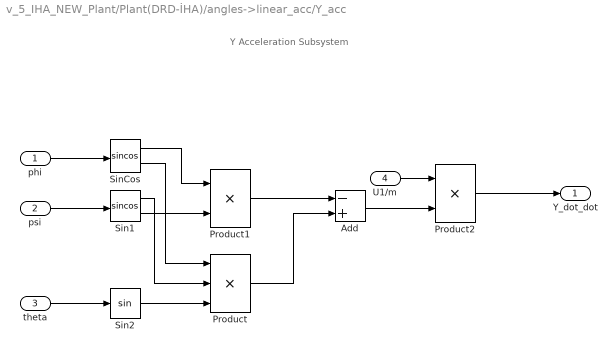
== system v_5_IHA_NEW_Plant/Plant(DRD-İHA)/angles->linear_acc/Y_acc ==
  note: Y Acceleration Subsystem
  phi : Inport
  psi : Inport  Port=2
  theta : Inport  Port=3
  U1/m : Inport  Port=4
  Add : Sum  Inputs=-+
  Product : Product  Inputs=3
  Product1 : Product
  Product2 : Product
  Sin1 : Trigonometry  Operator=sincos
  Sin2 : Trigonometry
  SinCos : Trigonometry  Operator=sincos
  "Y_dot_dot\t" : Outport
  wires:
  phi/1 -> SinCos/1
  psi/1 -> Sin1/1
  theta/1 -> Sin2/1
  Sin2/1 -> Product/3
  SinCos/1 -> Product1/1
  Product1/1 -> Add/1
  Product/1 -> Add/2
  Add/1 -> Product2/2
  Product2/1 -> "Y_dot_dot\t"/1
  U1/m/1 -> Product2/1
  SinCos/2 -> Product/1
  Sin1/1 -> Product/2
  Sin1/2 -> Product1/2

== system v_5_IHA_NEW_Plant/Plant(DRD-İHA)/angles->linear_acc/Z_acc ==
  note: Z Acceleration Subsystem
  phi : Inport
  theta : Inport  Port=2
  U1/m : Inport  Port=3
  Add : Sum  Inputs=-+
  Constant1 : Constant  Value=g
  Cos : Trigonometry  Operator=cos
  Product : Product  Inputs=3
  Sin1 : Trigonometry  Operator=cos
  "Z_dot_dot\t" : Outport
  wires:
  Sin1/1 -> Product/2
  Cos/1 -> Product/1
  Product/1 -> Add/2
  Constant1/1 -> Add/1
  phi/1 -> Sin1/1
  U1/m/1 -> Product/3
  theta/1 -> Cos/1
  Add/1 -> "Z_dot_dot\t"/1

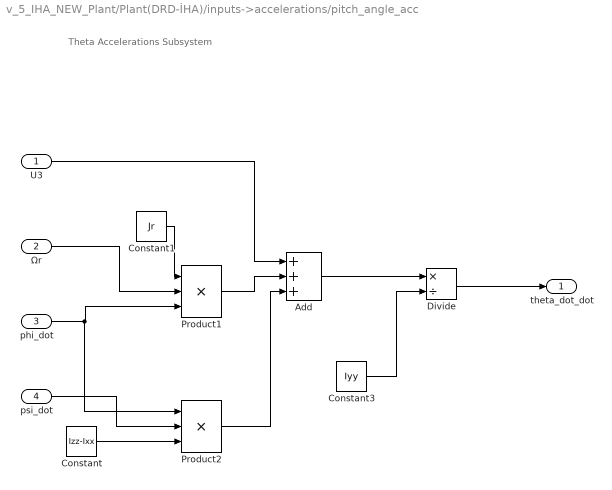
== system v_5_IHA_NEW_Plant/Plant(DRD-İHA)/inputs->accelerations/pitch_angle_acc ==
  note: Theta Accelerations Subsystem
  U3 : Inport
  Ωr : Inport  Port=2
  phi_dot : Inport  Port=3
  psi_dot : Inport  Port=4
  Add : Sum  Inputs=+++
  Constant : Constant  Value=Izz-Ixx
  Constant1 : Constant  Value=Jr
  Constant3 : Constant  Value=Iyy
  Divide : Product  Inputs=*/
  Product1 : Product  Inputs=3
  Product2 : Product  Inputs=3
  theta_dot_dot : Outport
  wires:
  Ωr/1 -> Product1/2
  phi_dot/1 -> Product2/1, Product1/3
  psi_dot/1 -> Product2/2
  Constant/1 -> Product2/3
  Constant1/1 -> Product1/1
  Product1/1 -> Add/2
  Product2/1 -> Add/3
  Add/1 -> Divide/1
  Constant3/1 -> Divide/2
  Divide/1 -> theta_dot_dot/1
  U3/1 -> Add/1

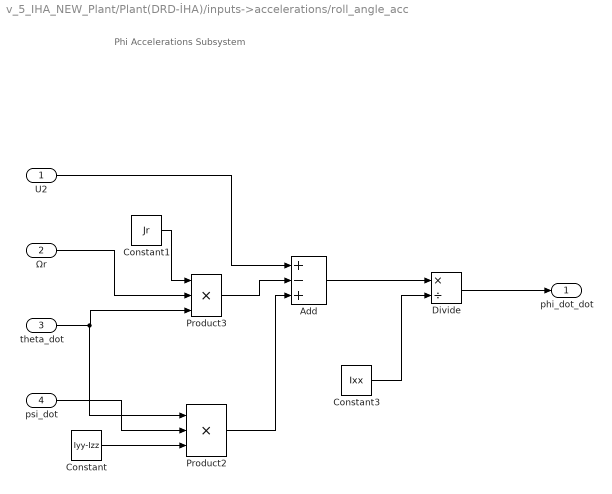
== system v_5_IHA_NEW_Plant/Plant(DRD-İHA)/inputs->accelerations/roll_angle_acc ==
  note: Phi Accelerations Subsystem
  U2 : Inport
  Ωr : Inport  Port=2
  theta_dot : Inport  Port=3
  psi_dot : Inport  Port=4
  Add : Sum  Inputs=+-+
  Constant : Constant  Value=Iyy-Izz
  Constant1 : Constant  Value=Jr
  Constant3 : Constant  Value=Ixx
  Divide : Product  Inputs=*/
  Product2 : Product  Inputs=3
  Product3 : Product  Inputs=3
  phi_dot_dot : Outport
  wires:
  Ωr/1 -> Product3/2
  theta_dot/1 -> Product3/3, Product2/1
  psi_dot/1 -> Product2/2
  Constant/1 -> Product2/3
  Constant1/1 -> Product3/1
  Product3/1 -> Add/2
  Product2/1 -> Add/3
  Add/1 -> Divide/1
  Constant3/1 -> Divide/2
  Divide/1 -> phi_dot_dot/1
  U2/1 -> Add/1

== system v_5_IHA_NEW_Plant/Plant(DRD-İHA)/inputs->accelerations/yaw_angle_acc ==
  note: Psi Accelerations Subsystem
  U4 : Inport
  theta_dot : Inport  Port=2
  phi_dot : Inport  Port=3
  Add : Sum
  Constant : Constant  Value=Ixx-Iyy
  Constant3 : Constant  Value=Izz
  Divide : Product  Inputs=*/
  Product1 : Product  Inputs=3
  psi_dot_dot : Outport
  wires:
  Product1/1 -> Add/2
  Add/1 -> Divide/1
  Constant3/1 -> Divide/2
  Divide/1 -> psi_dot_dot/1
  U4/1 -> Add/1
  theta_dot/1 -> Product1/1
  Constant/1 -> Product1/3
  phi_dot/1 -> Product1/2

== system v_5_IHA_NEW_Plant/Controller/PD and DQN Controller for Phi/DQN Controller for Phi/DQN Controller ==
  Z_error : Inport
  Z_actual : Inport  Port=2
  Exp : Math  Operator=reciprocal  SaturateOnIntegerOverflow=on
  Observation : Subsystem
  RL Agent : rllib/RL Agent  Agent=agent  ProvideReward=on  ProvideIsDone=on  ProvideCumRwd=off  TreatAsDirectFeedthrough=on  CollectLoggedSignals=on  CollectModelStates=on
  Reward : Subsystem
  Sum : Sum
  Theta_limit_penalty : Subsystem
  action : Outport
  wires:
  Exp/1 -> Reward/1(1/error)
  Observation/1(observation) -> RL Agent/1
  Theta_limit_penalty/1(reward) -> Sum/2
  Sum/1 -> RL Agent/2
  Reward/1(reward) -> Sum/1
  Theta_limit_penalty/2(stop) -> RL Agent/3
  RL Agent/1 -> action/1
  Z_actual/1 -> Observation/2("Theta_Actual ")
  Z_error/1 -> Observation/1(error), Theta_limit_penalty/1(error), Exp/1

== system v_5_IHA_NEW_Plant/Controller/PD and DQN Controller for Psi/DQN-DDPG Controller for Psi/DQN Controller ==
  Z_error : Inport
  Z_actual : Inport  Port=2
  Exp : Math  Operator=reciprocal  SaturateOnIntegerOverflow=on
  Observation : Subsystem
  RL Agent : rllib/RL Agent  Agent=agent  ProvideReward=on  ProvideIsDone=on  ProvideCumRwd=off  TreatAsDirectFeedthrough=on  CollectLoggedSignals=on  CollectModelStates=on
  Reward : Subsystem
  Sum : Sum
  Theta_limit_penalty : Subsystem
  action : Outport
  wires:
  Z_error/1 -> Exp/1, Theta_limit_penalty/1(error), Observation/1(error)
  Z_actual/1 -> Observation/2("Theta_Actual ")
  RL Agent/1 -> action/1
  Theta_limit_penalty/2(stop) -> RL Agent/3
  Reward/1(reward) -> Sum/1
  Sum/1 -> RL Agent/2
  Theta_limit_penalty/1(reward) -> Sum/2
  Observation/1(observation) -> RL Agent/1
  Exp/1 -> Reward/1(1/error)

== system v_5_IHA_NEW_Plant/Controller/PD and DQN Controller for Theta/DQN-DDPG Controller for Theta/DQN Controller ==
  Z_error : Inport
  Z_actual : Inport  Port=2
  Exp : Math  Operator=reciprocal  SaturateOnIntegerOverflow=on
  Observation : Subsystem
  RL Agent : rllib/RL Agent  Agent=agent  ProvideReward=on  ProvideIsDone=on  ProvideCumRwd=off  TreatAsDirectFeedthrough=on  CollectLoggedSignals=on  CollectModelStates=on
  Reward : Subsystem
  Sum : Sum
  Theta_limit_penalty : Subsystem
  action : Outport
  wires:
  Z_error/1 -> Exp/1, Theta_limit_penalty/1(error), Observation/1(error)
  Z_actual/1 -> Observation/2("Theta_Actual ")
  RL Agent/1 -> action/1
  Theta_limit_penalty/2(stop) -> RL Agent/3
  Reward/1(reward) -> Sum/1
  Sum/1 -> RL Agent/2
  Theta_limit_penalty/1(reward) -> Sum/2
  Observation/1(observation) -> RL Agent/1
  Exp/1 -> Reward/1(1/error)

== system v_5_IHA_NEW_Plant/Controller/PD and DQN-DDPG Controller for Z/DQN-DDPG Controller for Z/Observation ==
  error : Inport
  Actual_Z : Inport  Port=2
  Bus Creator : BusCreator  Inputs=4
  Derivative : Derivative
  Integrator : Integrator
  observation : Outport
  wires:
  error/1 -> Derivative/1, Integrator/1, Bus Creator/3
  Integrator/1 -> Bus Creator/1
  Derivative/1 -> Bus Creator/2
  Bus Creator/1 -> observation/1
  Actual_Z/1 -> Bus Creator/4

== system v_5_IHA_NEW_Plant/Controller/PD and DQN-DDPG Controller for Z/DQN-DDPG Controller for Z/Reward ==
  error : Inport
  Gain3 : Gain  Gain=-10
  Math Function : Math  Operator=square  SignedPower=on  SaturateOnIntegerOverflow=on
  reward : Outport  VectorParamsAs1DForOutWhenUnconnected=off
  wires:
  Gain3/1 -> reward/1
  error/1 -> Math Function/1
  Math Function/1 -> Gain3/1

== system v_5_IHA_NEW_Plant/Controller/PD and DQN-DDPG Controller for Z/DQN-DDPG Controller for Z/Theta_limit_penalty ==
  error : Inport
  Constant2 : Constant  Value=0
  Terminator : Terminator
  reward : Outport  VectorParamsAs1DForOutWhenUnconnected=off
  stop : Outport  Port=2  VectorParamsAs1DForOutWhenUnconnected=off
  wires:
  Constant2/1 -> stop/1, reward/1
  error/1 -> Terminator/1

== system v_5_IHA_NEW_Plant/Controller/PD and DQN Controller for Phi/DQN Controller for Phi/DQN Controller/Observation ==
  error : Inport
  "Theta_Actual " : Inport  Port=2
  Bus Creator : BusCreator  Inputs=3
  Discrete-Time Integrator : DiscreteIntegrator  SampleTime=Ts  ICPrevOutput=DiscIntNeverNeededParam  ICPrevScaledInput=DiscIntNeverNeededParam
  observation : Outport
  wires:
  error/1 -> Discrete-Time Integrator/1, Bus Creator/2
  Discrete-Time Integrator/1 -> Bus Creator/1
  "Theta_Actual "/1 -> Bus Creator/3
  Bus Creator/1 -> observation/1  "observation"

== system v_5_IHA_NEW_Plant/Controller/PD and DQN Controller for Phi/DQN Controller for Phi/DQN Controller/Reward ==
  1/error : Inport
  Gain1 : Gain  Commented=on  Gain=0.0001
  Gain3 : Gain  Gain=0.0001
  Math Function1 : Math  Operator=square  SignedPower=on  SaturateOnIntegerOverflow=on
  Math Function2 : Math  Commented=on  Operator=square  SignedPower=on  SaturateOnIntegerOverflow=on
  Square Root : Sqrt  SaturateOnIntegerOverflow=on
  Square Root1 : Sqrt  Commented=on  SaturateOnIntegerOverflow=on
  reward : Outport  VectorParamsAs1DForOutWhenUnconnected=off
  wires:
  Math Function2/1 -> Gain1/1
  Gain1/1 -> Square Root1/1
  Square Root/1 -> reward/1
  Gain3/1 -> Square Root/1
  1/error/1 -> Math Function1/1
  Math Function1/1 -> Gain3/1

== system v_5_IHA_NEW_Plant/Controller/PD and DQN Controller for Phi/DQN Controller for Phi/DQN Controller/Theta_limit_penalty ==
  error : Inport
  Abs : Abs
  Compare To Constant : simulink/Logic and Bit Operations/Compare To Constant  relop=>  const=15  OutDataTypeStr=boolean
  Gain1 : Gain  Gain=-10
  reward : Outport  VectorParamsAs1DForOutWhenUnconnected=off
  stop : Outport  Port=2  VectorParamsAs1DForOutWhenUnconnected=off
  wires:
  Gain1/1 -> reward/1
  Compare To Constant/1 -> Gain1/1, stop/1
  Abs/1 -> Compare To Constant/1
  error/1 -> Abs/1

== system v_5_IHA_NEW_Plant/Controller/PD and DQN Controller for Psi/DQN-DDPG Controller for Psi/DQN Controller/Observation ==
  error : Inport
  "Theta_Actual " : Inport  Port=2
  Bus Creator : BusCreator  Inputs=3
  Discrete-Time Integrator : DiscreteIntegrator  SampleTime=Ts  ICPrevOutput=DiscIntNeverNeededParam  ICPrevScaledInput=DiscIntNeverNeededParam
  observation : Outport
  wires:
  Bus Creator/1 -> observation/1  "observation"
  "Theta_Actual "/1 -> Bus Creator/3
  Discrete-Time Integrator/1 -> Bus Creator/1
  error/1 -> Bus Creator/2, Discrete-Time Integrator/1

== system v_5_IHA_NEW_Plant/Controller/PD and DQN Controller for Psi/DQN-DDPG Controller for Psi/DQN Controller/Reward ==
  1/error : Inport
  Gain1 : Gain  Commented=on  Gain=0.0001
  Gain3 : Gain  Gain=0.0001
  Math Function1 : Math  Operator=square  SignedPower=on  SaturateOnIntegerOverflow=on
  Math Function2 : Math  Commented=on  Operator=square  SignedPower=on  SaturateOnIntegerOverflow=on
  Square Root : Sqrt  SaturateOnIntegerOverflow=on
  Square Root1 : Sqrt  Commented=on  SaturateOnIntegerOverflow=on
  reward : Outport  VectorParamsAs1DForOutWhenUnconnected=off
  wires:
  Math Function1/1 -> Gain3/1
  1/error/1 -> Math Function1/1
  Gain3/1 -> Square Root/1
  Square Root/1 -> reward/1
  Gain1/1 -> Square Root1/1
  Math Function2/1 -> Gain1/1

== system v_5_IHA_NEW_Plant/Controller/PD and DQN Controller for Psi/DQN-DDPG Controller for Psi/DQN Controller/Theta_limit_penalty ==
  error : Inport
  Abs : Abs
  Compare To Constant : simulink/Logic and Bit Operations/Compare To Constant  relop=>  const=15  OutDataTypeStr=boolean
  Gain1 : Gain  Gain=-10
  reward : Outport  VectorParamsAs1DForOutWhenUnconnected=off
  stop : Outport  Port=2  VectorParamsAs1DForOutWhenUnconnected=off
  wires:
  error/1 -> Abs/1
  Abs/1 -> Compare To Constant/1
  Compare To Constant/1 -> stop/1, Gain1/1
  Gain1/1 -> reward/1

== system v_5_IHA_NEW_Plant/Controller/PD and DQN Controller for Theta/DQN-DDPG Controller for Theta/DQN Controller/Observation ==
  error : Inport
  "Theta_Actual " : Inport  Port=2
  Bus Creator : BusCreator  Inputs=3
  Discrete-Time Integrator : DiscreteIntegrator  SampleTime=Ts  ICPrevOutput=DiscIntNeverNeededParam  ICPrevScaledInput=DiscIntNeverNeededParam
  observation : Outport
  wires:
  Bus Creator/1 -> observation/1  "observation"
  "Theta_Actual "/1 -> Bus Creator/3
  Discrete-Time Integrator/1 -> Bus Creator/1
  error/1 -> Bus Creator/2, Discrete-Time Integrator/1

== system v_5_IHA_NEW_Plant/Controller/PD and DQN Controller for Theta/DQN-DDPG Controller for Theta/DQN Controller/Reward ==
  1/error : Inport
  Gain1 : Gain  Commented=on  Gain=0.0001
  Gain3 : Gain  Gain=0.0001
  Math Function1 : Math  Operator=square  SignedPower=on  SaturateOnIntegerOverflow=on
  Math Function2 : Math  Commented=on  Operator=square  SignedPower=on  SaturateOnIntegerOverflow=on
  Square Root : Sqrt  SaturateOnIntegerOverflow=on
  Square Root1 : Sqrt  Commented=on  SaturateOnIntegerOverflow=on
  reward : Outport  VectorParamsAs1DForOutWhenUnconnected=off
  wires:
  Math Function1/1 -> Gain3/1
  1/error/1 -> Math Function1/1
  Gain3/1 -> Square Root/1
  Square Root/1 -> reward/1
  Gain1/1 -> Square Root1/1
  Math Function2/1 -> Gain1/1

== system v_5_IHA_NEW_Plant/Controller/PD and DQN Controller for Theta/DQN-DDPG Controller for Theta/DQN Controller/Theta_limit_penalty ==
  error : Inport
  Abs : Abs
  Compare To Constant : simulink/Logic and Bit Operations/Compare To Constant  relop=>  const=15  OutDataTypeStr=boolean
  Gain1 : Gain  Gain=-10
  reward : Outport  VectorParamsAs1DForOutWhenUnconnected=off
  stop : Outport  Port=2  VectorParamsAs1DForOutWhenUnconnected=off
  wires:
  error/1 -> Abs/1
  Abs/1 -> Compare To Constant/1
  Compare To Constant/1 -> stop/1, Gain1/1
  Gain1/1 -> reward/1

== matlab function v_5_IHA_NEW_Plant/Scope/array2array ==
  data: array_desired input; X_array output; array_out input; Y_array output; Z_array output; Phi_array output; Theta_array output; Psi_array output
function [X_array,Y_array,Z_array,Phi_array,Theta_array,Psi_array] = array2array(array_desired,array_out)
X = array_out(1);
Y = array_out(2);
Z = array_out(3);
Phi = array_out(4);
Theta = array_out(5);
Psi = array_out(6);

Z_d = array_desired(1);
Phi_d = array_desired(2);
Theta_d = array_desired(3);
Psi_d = array_desired(4);

X_array=[X];
Y_array=[Y];
Z_array=[Z Z_d];
Phi_array=[Phi Phi_d];
Theta_array=[Theta Theta_d];
Psi_array=[Psi Psi_d]; 

end

== matlab function v_5_IHA_NEW_Plant/IAE Subsystem/IAE for Z/error2abs ==
  data: error input; abs output
function abs = error2abs(error)
    if(error<0)
        error = error*(-1);
    end
abs = error;
end

== matlab function v_5_IHA_NEW_Plant/IAE Subsystem/IAE for Phi/error2abs ==
  data: error input; abs output
function abs = error2abs(error)
    if(error<0)
        error = error*(-1);
    end
abs = error;
end

== matlab function v_5_IHA_NEW_Plant/IAE Subsystem/IAE for Theta/error2abs ==
  data: error input; abs output
function abs = error2abs(error)
    if(error<0)
        error = error*(-1);
    end
abs = error;
end

== matlab function v_5_IHA_NEW_Plant/IAE Subsystem/IAE for Psi/error2abs ==
  data: error input; abs output
function abs = error2abs(error)
    if(error<0)
        error = error*(-1);
    end
abs = error;
end

== matlab function v_5_IHA_NEW_Plant/Plant(DRD-İHA)/Omega_Calculate /saturation ==
  data: upper input; input input; input output; lower input
function input = saturation(upper,input,lower)

    if(input > upper)
        input = upper;
    elseif(input < lower)
        input = lower;
    end

end

== matlab function v_5_IHA_NEW_Plant/Plant(DRD-İHA)/Omega_Calculate /saturation1 ==
  data: upper input; input input; input output; lower input
function input = saturation(upper,input,lower)

    if(input > upper)
        input = upper;
    elseif(input < lower)
        input = lower;
    end

end

== matlab function v_5_IHA_NEW_Plant/Plant(DRD-İHA)/Omega_Calculate /saturation2 ==
  data: upper input; input input; input output; lower input
function input = saturation(upper,input,lower)

    if(input > upper)
        input = upper;
    elseif(input < lower)
        input = lower;
    end

end

== matlab function v_5_IHA_NEW_Plant/Plant(DRD-İHA)/Omega_Calculate /saturation3 ==
  data: upper input; input input; input output; lower input
function input = saturation(upper,input,lower)

    if(input > upper)
        input = upper;
    elseif(input < lower)
        input = lower;
    end

end
